simulink model "problem_8"  (R2020a)
settings: Solver=VariableStepAuto  StartTime=0.0  StopTime=10.0  RelTol=1e-3
settings Model: Creator=USER  LastModifiedBy=USER

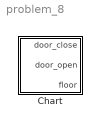
== system problem_8 ==
  Chart : Stateflow chart  TreatAsAtomicUnit=on

== stateflow chart problem_8/Chart ==
  state LiftControl [parallel]
    settings: executionOrder=1
    state Hall
    state LiftOperation
      en:door_open=1;
      state Normal
      state LiftUp
        en:count=0;
        during:
        count=count+1;
      state LiftDown
        en:count=0;
        during:
        count=count+1;
      (default) -> Normal
      Normal -> LiftDown [order 2] : {send(DOWN,liftUpDown);}
      Normal -> LiftUp [order 1] : {send(UP,liftUpDown);}
      LiftUp -> Normal : [count>3]
      LiftDown -> Normal : [count>3]
    (default) -> Hall
    Hall -> LiftOperation
  state liftUpDown [parallel]
    settings: executionOrder=2
    state Floor4
      en:floor=4;
      during:door_open=0;
      door_close=1;
      exit:door_open=1;
    state Floor2
      en:floor=2;
      during:door_open=0;
      door_close=1;
      exit:door_open=1;
    state Floor3
      en:floor=3;
      during:door_open=0;
      door_close=1;
      exit:door_open=1;
    state Floor5
      floor=5;
      during:door_open=0;
      door_close=1;
      exit:door_open=1;
    state Floor1
      en:floor=1;
      during:door_open=0;
      door_close=1;
      exit:door_open=1;
    (default) -> Floor1
    Floor3 -> Floor4 [order 1] : UP
    Floor2 -> Floor3 [order 1] : UP
    Floor4 -> Floor5 [order 1] : UP
    Floor1 -> Floor2 : UP
    Floor4 -> Floor3 [order 2] : DOWN
    Floor3 -> Floor2 [order 2] : DOWN
    Floor5 -> Floor4 : DOWN
    Floor2 -> Floor1 [order 2] : DOWN
  data: door_close output; door_open output; floor output; count local
  events: DOWN local RISING_EDGE_EVENT; UP local RISING_EDGE_EVENT
